simulink model "task_4"  (Simulink 7.6)
settings: Solver=ode45  StartTime=0.0  StopTime=0.3  RelTol=1e-3
settings Model: Creator=Admin  LastModifiedBy=Admin

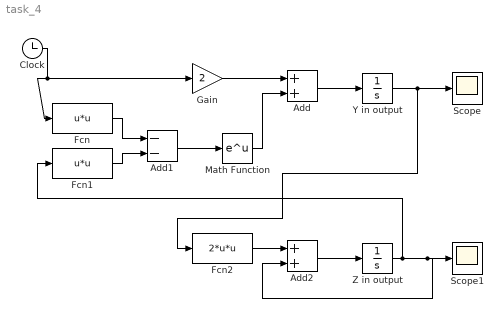
== system task_4 ==
  Add : Sum
  Add1 : Sum  Inputs=--
  Add2 : Sum
  Clock : Clock
      settings: Decimation=10
  Fcn : Fcn  Expr=u*u
  Fcn1 : Fcn  Expr=u*u
  Fcn2 : Fcn  Expr=2*u*u
  Gain : Gain  Gain=2
  Math Function : Math  SaturateOnIntegerOverflow=on
  Scope : Scope
  Scope1 : Scope
  Y in output : Integrator  InitialCondition=0.5
  Z in output : Integrator  InitialCondition=1
  wires:
  Add/1 -> Y in output/1
  Clock/1 -> Gain/1, Fcn/1
  Gain/1 -> Add/1
  Math Function/1 -> Add/2
  Add1/1 -> Math Function/1
  Z in output/1 -> Fcn1/1, Add2/2, Scope1/1
  Fcn/1 -> Add1/1
  Fcn1/1 -> Add1/2
  Add2/1 -> Z in output/1
  Fcn2/1 -> Add2/1
  Y in output/1 -> Fcn2/1, Scope/1
